simulink model "H_inf_synth_model"  (R2024a)
settings: Solver=VariableStepAuto  StartTime=0.0  StopTime=2000  RelTol=1e-3
libraries: cstblocks x6
settings Model: Creator=Denis  LastModifiedBy=denisroutkevitch
settings OptimizationCC: ReuseModelBlockBuffer=off
settings RTWCC: GPUComputeCapability=3.5

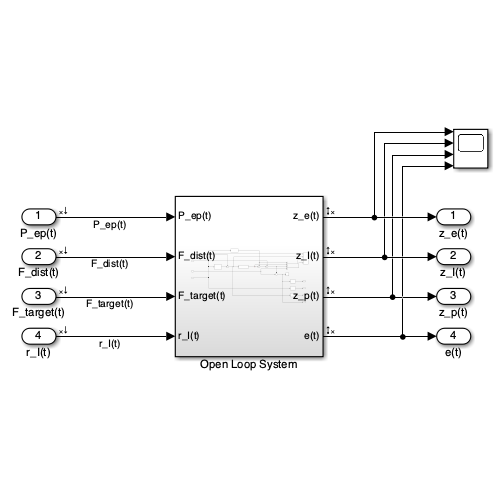
[thumbnail: Simulink's stored preview of the top-level diagram]
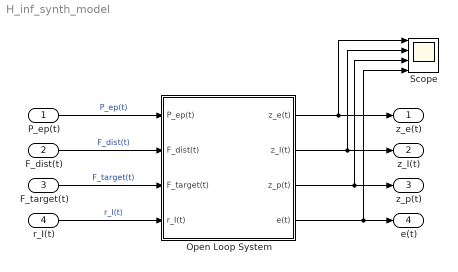
== system H_inf_synth_model ==
  P_ep(t) : Inport
  F_dist(t) : Inport  Port=2
  F_target(t) : Inport  Port=3
  r_I(t) : Inport  Port=4
  Open Loop System : Subsystem
  Scope : Scope  NumInputPorts=4
  z_e(t) : Outport
  z_I(t) : Outport  Port=2
  z_p(t) : Outport  Port=3
  e(t) : Outport  Port=4
  wires:
  P_ep(t)/1 -> Open Loop System/1(P_ep(t))  "P_ep(t)"
  Open Loop System/1(z_e(t)) -> z_e(t)/1, Scope/1
  Open Loop System/3(z_p(t)) -> z_p(t)/1, Scope/3
  Open Loop System/2(z_I(t)) -> z_I(t)/1, Scope/2
  F_target(t)/1 -> Open Loop System/3(F_target(t))  "F_target(t)"
  Open Loop System/4(e(t)) -> e(t)/1, Scope/4
  r_I(t)/1 -> Open Loop System/4(r_I(t))  "r_I(t)"
  F_dist(t)/1 -> Open Loop System/2(F_dist(t))  "F_dist(t)"

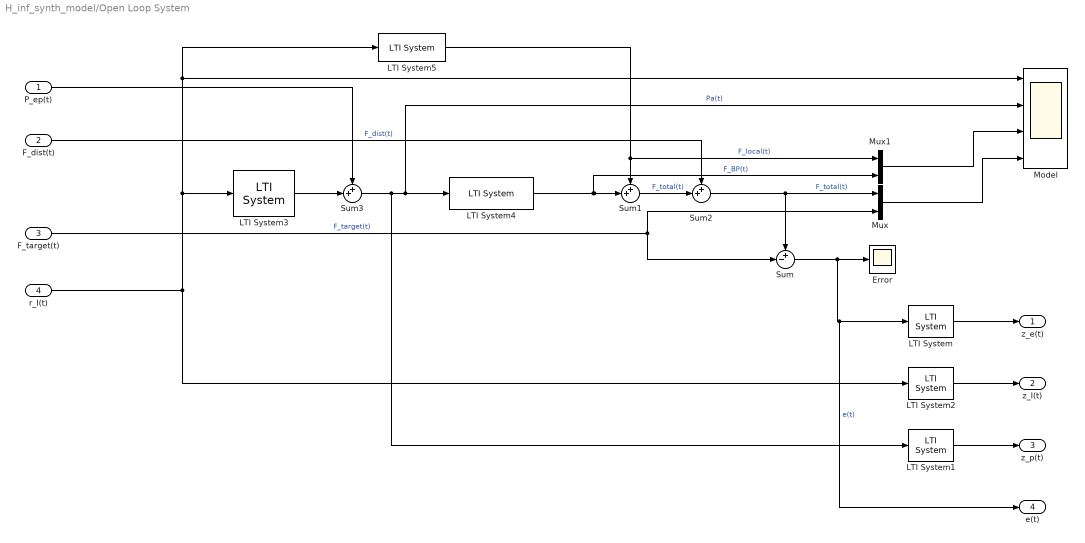
== system H_inf_synth_model/Open Loop System ==
  P_ep(t) : Inport
  F_dist(t) : Inport  Port=2
  F_target(t) : Inport  Port=3
  r_I(t) : Inport  Port=4
  Error : Scope
  LTI System : cstblocks/LTI System  sys=W_e  IC=[]  PadeOrder=0
  LTI System1 : cstblocks/LTI System  sys=W_p  IC=[]  PadeOrder=0
  LTI System2 : cstblocks/LTI System  sys=W_I  IC=[]  PadeOrder=0
  LTI System3 : cstblocks/LTI System  sys=H_IP_d  IC=[]  PadeOrder=0
  LTI System4 : cstblocks/LTI System  sys=H_PF_inj  IC=[]  PadeOrder=0
  LTI System5 : cstblocks/LTI System  sys=H_IF_d  IC=[]  PadeOrder=0
  Model : Scope  NumInputPorts=4
  Mux : Mux  Inputs=2
  Mux1 : Mux  Inputs=2
  Sum : Sum  Inputs=+-|
  Sum1 : Sum  Inputs=++|
  Sum2 : Sum  Inputs=++|
  Sum3 : Sum  Inputs=++|
  z_e(t) : Outport
  z_I(t) : Outport  Port=2
  z_p(t) : Outport  Port=3
  e(t) : Outport  Port=4
  wires:
  Sum3/1 -> LTI System1/1, Model/2, LTI System4/1  "Pa(t)"
  LTI System4/1 -> Sum1/2, Mux1/2  "F_BP(t)"
  LTI System5/1 -> Sum1/1, Mux1/1  "F_local(t)"
  Sum/1 -> e(t)/1, LTI System/1, Error/1  "e(t)"
  P_ep(t)/1 -> Sum3/1
  r_I(t)/1 -> LTI System2/1, LTI System3/1, LTI System5/1, Model/1
  Mux1/1 -> Model/3
  Sum2/1 -> Sum/1, Mux/1  "F_total(t)"
  Mux/1 -> Model/4
  LTI System3/1 -> Sum3/2
  F_target(t)/1 -> Sum/2, Mux/2  "F_target(t)"
  LTI System2/1 -> z_I(t)/1
  LTI System/1 -> z_e(t)/1
  LTI System1/1 -> z_p(t)/1
  F_dist(t)/1 -> Sum2/1  "F_dist(t)"
  Sum1/1 -> Sum2/2  "F_total(t)"
